simulink model "StateFlow_varB"  (R2022b)
settings: Solver=VariableStepAuto  StartTime=0.0  StopTime=500  FixedStep=0.001  RelTol=1e-3
InitFcn:
  | State_Flow_varB_setting
values from neighbouring files (symbols this model uses):
  Acceptable_press_offset = 5    [State_Flow_varB_setting.m]
  Desired_pressure_in_oxidiser_tank = 40    [State_Flow_varB_setting.m]
  Desired_pressure_in_pressure_section1 = 150    [State_Flow_varB_setting.m]
  Desired_pressure_in_pressure_section2 = 180    [State_Flow_varB_setting.m]
  s = struct    [State_Flow_varB_setting.m]
  Servo_open_limit = 20    [State_Flow_varB_setting.m]
  UDP_FC_send_packet_length = 68    [State_Flow_varB_setting.m]
  UDP_FC_send_sample_time = 0.05    [State_Flow_varB_setting.m]
  UDP_GSE_Curr_loop_receive_sample_time = 0.01    [State_Flow_varB_setting.m]
  UDP_GSE_IO_send_sample_time = 0.05    [State_Flow_varB_setting.m]
  UDP_GSE_send_packet_length = 68    [State_Flow_varB_setting.m]
libraries: simulink x36, slrealtimeiplib x16, slpidlib x6
(part 3 of 3)

== matlab function StateFlow_varB/Subsystem6/Subsystem3/Subsystem1/MATLAB Function1 ==
  data: data_new input; y output; data_prev input double; workspace input
function y = fcn(data_new, data_prev, workspace)

coder.extrinsic('set_param')
%disp(data_prev(2))
press_sensor100bar_conv = @(x) workspace.PT5302_GAIN*double(x) + workspace.PT5302_OFFSET;
press_sensor300bar_conv = @(x) workspace.PT5500_GAIN*double(x) + workspace.PT5500_OFFSET;
output_format = @(Fill_N2_state, ...
                  Release_N2_state, ...
                  Fill_N2O_state, ...
                  Release_N2O_state, ...
                  Servo_0_state, ...
                  Servo_1_state, ...
                  N2_tank_pressure, ...
                  N2_bomb_pressure, ...
                  N2O_tank_pressure, ...
                  N2O_bomb_pressure, ...
                  N2O_fuel_level_sensor) [Fill_N2_state, Release_N2_state, Fill_N2O_state, Release_N2O_state, Servo_0_state, Servo_1_state, N2_tank_pressure, N2_bomb_pressure, N2O_tank_pressure, N2O_bomb_pressure, N2O_fuel_level_sensor];


y = output_format(0,0,0,0,0,0,0,0,0,0,0);

data_n = typecast(data_new,'uint8');
id = data_n(1);
pl = data_n(2);
msg_id = data_n(3);
card_id = data_n(4);
slot = data_n(5);
message = data_n(6:end);

switch card_id
    case workspace.CARDID_CURRENT_LOOP
        message_CUL = typecast(message, 'uint32');
        %disp(message_CUL.');
        %disp('---------------------------------------')
        low_p = message_CUL(workspace.Low_p_ind);                                   %N2O tank inside rocket
        high_p = message_CUL(workspace.High_p_ind);                                 %N2 tank inside rocket
        GSE_oxidiser_p = message_CUL(workspace.GSE_oxidiser_p_ind);                 %N2O tank outside rocket
        GSE_Pressurizer_p = message_CUL(workspace.GSE_Pressurizer_p_ind);           %N2 tank outside rocket
        N2O_fuel_level = double(message_CUL(workspace.N2O_fuel_level_ind));                 %probably needst to be modified
        
        low_p_bar = press_sensor100bar_conv(low_p);
        high_p_bar = press_sensor300bar_conv(high_p);
        GSE_oxidiser_bar = press_sensor300bar_conv(GSE_oxidiser_p);
        GSE_Pressurizer_bar = press_sensor300bar_conv(GSE_Pressurizer_p);
        y = output_format(data_prev(1), data_prev(2), data_prev(3), data_prev(4), data_prev(5), data_prev(6), high_p_bar, GSE_Pressurizer_bar, low_p_bar, GSE_oxidiser_bar, N2O_fuel_level);
    case workspace.CARDID_IO
        switch slot
            case workspace.CARD_IO1_SLOT
                y = output_format(data_prev(1), data_prev(2), data_prev(3), data_prev(4), data_prev(5), data_prev(6), data_prev(7), data_prev(8), data_prev(9), data_prev(10), data_prev(11)); 
            case workspace.CARD_IO2_SLOT
                message_CIO2 = typecast(message, 'uint8');
                
                %Fault state check
                if message_CIO2(workspace.H0_bridge_fault_state_ind) == workspace.H_bridge_fault_state_num 
                    set_param('StateFlow_varB/Subsystem6/Subsystem3/Constant6', 'Value', '0')
                else
                    set_param('StateFlow_varB/Subsystem6/Subsystem3/Constant6', 'Value', '1')
                end

                if message_CIO2(workspace.H1_bridge_fault_state_ind) == workspace.H_bridge_fault_state_num 
                    set_param('StateFlow_varB/Subsystem6/Subsystem3/Constant8', 'Value', '0')
                else
                    set_param('StateFlow_varB/Subsystem6/Subsystem3/Constant8', 'Value', '1')
                end

                if message_CIO2(workspace.H2_bridge_fault_state_ind) == workspace.H_bridge_fault_state_num 
                    set_param('StateFlow_varB/Subsystem6/Subsystem3/Constant9', 'Value', '0')
                else
                    set_param('StateFlow_varB/Subsystem6/Subsystem3/Constant9', 'Value', '1')
                end
                
                Fill_bridge_state_N2 = double(message_CIO2(workspace.H1_bridge_state_ind));
                Fill_bridge_state_N2O = double(message_CIO2(workspace.H2_bridge_state_ind));
                Servo_0_state = double(message_CIO2(workspace.Servo_0_state_ind));
                Servo_1_state = double(message_CIO2(workspace.Servo_1_state_ind));

                if Servo_0_state >= 10
                    set_param('StateFlow_varB/Subsystem6/Subsystem3/Constant2', 'Value', '1')
                else
                    set_param('StateFlow_varB/Subsystem6/Subsystem3/Constant2', 'Value', '0')
                end

                if Servo_1_state >= 10
                    set_param('StateFlow_varB/Subsystem6/Subsystem3/Constant3', 'Value', '1')
                else
                    set_param('StateFlow_varB/Subsystem6/Subsystem3/Constant3', 'Value', '0')
                end

                y = output_format(Fill_bridge_state_N2, data_prev(2), Fill_bridge_state_N2O, data_prev(4), Servo_0_state, Servo_1_state, data_prev(7), data_prev(8), data_prev(9), data_prev(10), data_prev(11)); 
            case workspace.CARD_IO3_SLOT
                message_CIO3 = typecast(message, 'uint8');
                
                %Fault state check
                if message_CIO3(workspace.H0_bridge_fault_state_ind) == workspace.H_bridge_fault_state_num 
                    set_param('StateFlow_varB/Subsystem6/Subsystem3/Constant10', 'Value', '0') %needs to be changed to 0
                else
                    set_param('StateFlow_varB/Subsystem6/Subsystem3/Constant10', 'Value', '1')
                end
                

                if message_CIO3(workspace.H1_bridge_fault_state_ind) == workspace.H_bridge_fault_state_num  
                    set_param('StateFlow_varB/Subsystem6/Subsystem3/Constant11', 'Value', '0') 
                else
                    set_param('StateFlow_varB/Subsystem6/Subsystem3/Constant11', 'Value', '1')
                end

                if message_CIO3(workspace.H2_bridge_fault_state_ind) == workspace.H_bridge_fault_state_num 
                    set_param('StateFlow_varB/Subsystem6/Subsystem3/Constant12', 'Value', '0')
                else
                    set_param('StateFlow_varB/Subsystem6/Subsystem3/Constant12', 'Value', '1')
                end
                
                Release_bridge_state_N2 = double(message_CIO3(workspace.H1_bridge_state_ind));
                Release_bridge_state_N2O = double(message_CIO3(workspace.H2_bridge_state_ind));

                if Release_bridge_state_N2 ~= 0
                    set_param('StateFlow_varB/Subsystem6/Subsystem3/Constant5', 'Value', '1')
                else
                    set_param('StateFlow_varB/Subsystem6/Subsystem3/Constant5', 'Value', '0')
                end

                y = output_format(data_prev(1), Release_bridge_state_N2, data_prev(3), Release_bridge_state_N2O, data_prev(5), data_prev(6), data_prev(7), data_prev(8), data_prev(9), data_prev(10), data_prev(11)); 
            otherwise
                y = output_format(data_prev(1), data_prev(2), data_prev(3), data_prev(4), data_prev(5), data_prev(6), data_prev(7), data_prev(8), data_prev(9), data_prev(10), data_prev(11)); 
        end

    otherwise 
        y = output_format(data_prev(1), data_prev(2), data_prev(3), data_prev(4), data_prev(5), data_prev(6), data_prev(7), data_prev(8), data_prev(9), data_prev(10), data_prev(11)); 
end

end

== matlab function StateFlow_varB/Subsystem6/Subsystem3/MATLAB Function1 ==
  data: val_const input; valves_state input; workspace input; u input; y output

function y = fcn(val_const, valves_state, workspace, u)

coder.extrinsic('set_param')

if u >= val_const
    set_param('StateFlow_varB/Subsystem6/Subsystem3/Constant1', 'Value', sprintf('%f',u))
    y = 0;
else
   first_valve = valves_state(3);
   second_valve = valves_state(2);
   if ~(first_valve || second_valve)
       if u <= (val_const - workspace.Pressure_drop_const)
           set_param('StateFlow_varB/Subsystem6/Constant', 'Value', '0')
           y = 1;
       else
           y = 0;
       end
   else
       set_param('StateFlow_varB/Subsystem6/Subsystem3/Constant1', 'Value', sprintf('%f',u))
       y = 0;
   end
end

end

== matlab function StateFlow_varB/Subsystem6/Subsystem10/MATLAB Function6 ==
  data: u1 input; u2 input; u3 input; u4 input; y output; cntr_prev input; cntr output
function [y, cntr] = fcn(u1, u2, u3, u4, cntr_prev)

y = uint8(zeros(1,68));

switch cntr_prev
    case 1
        y = u1;
    case 2
        y = u2;
    case 3
        y = u3;
    case 4
        y = u4;
end

if cntr_prev < 4
    cntr = cntr_prev + 1;
else
    cntr = 1;
end

== matlab function StateFlow_varB/Subsystem6/Subsystem10/MATLAB Function7 ==
  data: u1 input; u2 input; y output; cntr_prev input; cntr output
function [y, cntr] = fcn(u1, u2, cntr_prev)


y = uint8(zeros(1,68));

switch cntr_prev
    case 1
        y = u1;
    case 2
        y = u2;
end

if cntr_prev < 2
    cntr = cntr_prev + 1;
else
    cntr = 1;
end

== matlab function StateFlow_varB/Subsystem6/Subsystem/Subsystem2/Subsystem6/MATLAB Function6 ==
  data: u1 input; u2 input; y output; cntr_prev input; cntr output
function [y, cntr] = fcn(u1, u2, cntr_prev)


y = uint8(zeros(1,68));

switch cntr_prev
    case 1
        y = u1;
    case 2
        y = u2;
end

if cntr_prev < 2
    cntr = cntr_prev + 1;
else
    cntr = 1;
end

== matlab function StateFlow_varB/Subsystem6/Subsystem/Subsystem2/Subsystem7/MATLAB Function6 ==
  data: u1 input; u2 input; u3 input; y output; cntr_prev input; cntr output
function [y, cntr] = fcn(u1, u2, u3, cntr_prev)


y = uint8(zeros(1,68));

switch cntr_prev
    case 1
        y = u1;
    case 2
        y = u2;
    case 3
        y = u3;
end

if cntr_prev < 3
    cntr = cntr_prev + 1;
else
    cntr = 1;
end

== matlab function StateFlow_varB/Subsystem6/Subsystem/Subsystem2/Subsystem9/MATLAB Function6 ==
  data: u1 input; u2 input; length input; y output size=[1,68]; cntr_prev input; cntr output
function [y, cntr] = fcn(u1, u2, length, cntr_prev)


y = uint8(zeros(1,68));

switch cntr_prev
    case 1
        y = u1;
    case 2
        y = u2;
end

if cntr_prev < 2
    cntr = cntr_prev + 1;
else
    cntr = 1;
end

== matlab function StateFlow_varB/Subsystem6/Subsystem/Subsystem2/Subsystem10/MATLAB Function6 ==
  data: u1 input; u2 input; u3 input; u4 input; y output; cntr_prev input; cntr output
function [y, cntr] = fcn(u1, u2, u3, u4, cntr_prev)


y = uint8(zeros(1,68));

switch cntr_prev
    case 1
        y = u1;
    case 2
        y = u2;
    case 3
        y = u3;
    case 4
        y = u4;
end

if cntr_prev < 4
    cntr = cntr_prev + 1;
else
    cntr = 1;
end

== matlab function StateFlow_varB/Subsystem6/Subsystem2/MATLAB Function ==
  data: valve input; time_curr output; time_des input; time_curr1 input
function time_curr = fcn(valve, time_des, time_curr1)

coder.extrinsic("set_param")

if (time_des - time_curr1) <= 0
    switch valve
        case 0
            set_param('StateFlow_varB/Subsystem6/Subsystem10/Constant9', 'Value', '0');
        case 1
            set_param('StateFlow_varB/Subsystem6/Subsystem10/Constant10', 'Value', '0');
        case 2
            set_param('StateFlow_varB/Subsystem6/Subsystem10/Constant13', 'Value', '0');
        case 3
            set_param('StateFlow_varB/Subsystem6/Subsystem10/Constant14', 'Value', '0');
        case 4
            set_param('StateFlow_varB/Subsystem6/Subsystem10/Constant11', 'Value', '0');
        case 5
            set_param('StateFlow_varB/Subsystem6/Subsystem10/Constant12', 'Value', '0');
    end
    set_param('StateFlow_varB/Subsystem6/Constant1', 'Value', '0');
else
    switch valve
        case 0
            set_param('StateFlow_varB/Subsystem6/Subsystem10/Constant9', 'Value', '1');
        case 1
            set_param('StateFlow_varB/Subsystem6/Subsystem10/Constant10', 'Value', '1');
        case 2
            set_param('StateFlow_varB/Subsystem6/Subsystem10/Constant13', 'Value', '1');
        case 3
            set_param('StateFlow_varB/Subsystem6/Subsystem10/Constant14', 'Value', '1');
        case 4
            set_param('StateFlow_varB/Subsystem6/Subsystem10/Constant11', 'Value', '1');
        case 5
            set_param('StateFlow_varB/Subsystem6/Subsystem10/Constant12', 'Value', '1');
    end
end    

time_curr = time_curr1 + 0.05;

== matlab function StateFlow_varB/Subsystem6/Subsystem3/MATLAB Function2 ==
  data: H0_IO2 input; H1_IO2 input; H2_IO2 input; H0_IO3 input; H1_IO3 input; H2_IO3 input
function fcn(H0_IO2, H1_IO2, H2_IO2, H0_IO3, H1_IO3, H2_IO3)

coder.extrinsic("set_param")

if H0_IO2 == 0 || H1_IO2 == 0 || H2_IO2 == 0 || H0_IO3 == 0 || H1_IO3 == 0 || H2_IO3 == 0
     set_param('StateFlow_varB/Subsystem6/Constant', 'Value', '0')
end

== matlab function StateFlow_varB/Subsystem6/Subsystem/Subsystem9/MATLAB Function2 ==
  data: u input; cntr input; fill output; release output; workspace input; duty output; previous_duty input
function [fill, release, duty]= fcn(u, ...
                                    cntr, ...
                                    workspace, ...
                                    previous_duty)

%Halving duty cycle
duty = previous_duty;
if cntr
    duty = previous_duty / 2;
end

%Deciding which valve should be open
if u > workspace.Acceptable_press_offset
    fill = duty;
    release = 0;
elseif u < -workspace.Acceptable_press_offset
    release = duty;
    fill = 0;
else
    fill = 0;
    release = 0;
end

== matlab function StateFlow_varB/Subsystem6/Subsystem/Subsystem2/Subsystem7/MATLAB Function3 ==
  data: input input; code output; workspace input
function code = fcn(input, workspace)

if input == 1
    code = workspace.N2O_fill_valve_open;
else
    code = workspace.N2O_fill_valve_close;
end

end

== matlab function StateFlow_varB/Subsystem6/Subsystem/Subsystem18/MATLAB Function2 ==
  data: u input; cntr input; fill output; release output; workspace input; duty output; previous_duty input
function [fill, release, duty]= fcn(u, ...
                                    cntr, ...
                                    workspace, ...
                                    previous_duty)

%Halving duty cycle
duty = previous_duty;
if cntr
    duty = previous_duty / 2;
end

%Deciding which valve should be open
if u > workspace.Acceptable_press_offset
    fill = duty;
    release = 0;
elseif u < -workspace.Acceptable_press_offset
    release = duty;
    fill = 0;
else
    fill = 0;
    release = 0;
end

== matlab function StateFlow_varB/Subsystem6/Subsystem/Subsystem13/MATLAB Function2 ==
  data: u input; cntr input; fill output; release output; workspace input; duty output; previous_duty input
function [fill, release, duty]= fcn(u, ...
                                    cntr, ...
                                    workspace, ...
                                    previous_duty)

%Halving duty cycle
duty = previous_duty;
if cntr
    duty = previous_duty / 2;
end

%Deciding which valve should be open
if u > 5
    fill = duty;
    release = 0;
elseif u < -5
    release = duty;
    fill = 0;
else
    fill = 0;
    release = 0;
end
